simulink model "LHC_18kW_v0"  (R2015a)
settings: Solver=ode15s  StartTime=0.0  StopTime=10000  RelTol=1e-3
libraries: simCryogenics_lib x24, nesl_utility x16
settings Model: Creator=SK248285  LastModifiedBy=FB229602
settings SimscapeCC: SimscapeLogType=all  SimscapeLogLimitData=off

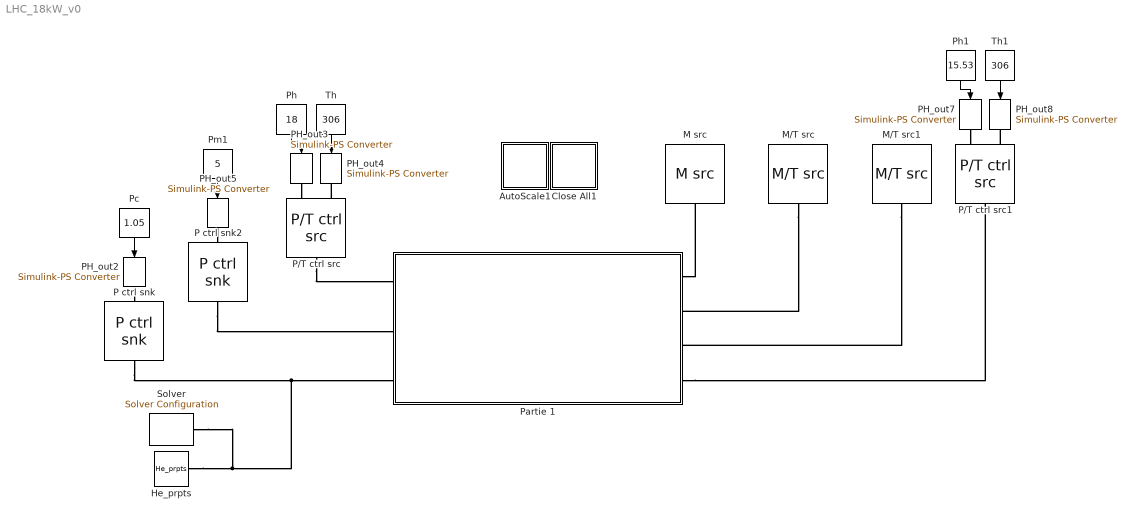
== system LHC_18kW_v0 ==
  AutoScale1 : Subsystem
      settings: OpenFcn=|
      | set(0, 'showhiddenhandles', 'on')
      | 
      | scope = findobj(0, 'Tag', 'SIMULINK_SIMSCOPE_FIGURE');
      | 
      | for i=1:length(scope)
      |   simscope('ScopeBar', 'ActionIcon', 'Find',     scope(i))
      | end
      | 
      | set(0, 'showhiddenhandles', 'off')
      mask Display: disp('Auto\nScale\nScope')
  Close All1 : Subsystem
      settings: OpenFcn=|
      | set(0, 'showhiddenhandles', 'on')
      | scope = findobj(0, 'Tag','SIMULINK_SIMSCOPE_FIGURE');
      | close(scope)
      | set(0, 'showhiddenhandles', 'off')
      mask Display: disp('Close\nAll\nScope')
  He_prpts : simCryogenics_lib/Utilities/He_prpts  P_min=0.1 bar  T_min=50 K  T_max=320 K  P_max=20 bar  Mol=4.0026 * 10 ^ (- 3) kg/mol
  M src : simCryogenics_lib/Sources_Sinks/M src  M=1 kg/s
  M/T src : simCryogenics_lib/Sources_Sinks/M//T src  M=0.350 kg/s  T=89 K
  M/T src1 : simCryogenics_lib/Sources_Sinks/M//T src  M=0.650 kg/s  T=89 K
  P ctrl snk : simCryogenics_lib/Sources_Sinks/P ctrl snk
  P ctrl snk2 : simCryogenics_lib/Sources_Sinks/P ctrl snk
  P/T ctrl src : simCryogenics_lib/Sources_Sinks/P//T ctrl src
  P/T ctrl src1 : simCryogenics_lib/Sources_Sinks/P//T ctrl src
  PH_out{2..3,5,7} (4 alike) : nesl_utility/Simulink-PS Converter  PhysicalDomain=network_engine_domain  SubClassName=ps_input  LeftPortType=input  RightPortType=output  PseudoPeriodic=off  Frequencies=[]  NoiseDistribution=none  NoiseParameters=[]  Unit=bar  AffineConversion=off  InputFiltering=off  SimscapeFilterOrder=1  InputFilterTimeConstant=0.001  UdotUserProvided=1
  PH_out4 : nesl_utility/Simulink-PS Converter  PhysicalDomain=network_engine_domain  SubClassName=ps_input  LeftPortType=input  RightPortType=output  PseudoPeriodic=off  Frequencies=[]  NoiseDistribution=none  NoiseParameters=[]  Unit=K  AffineConversion=off  InputFiltering=off  SimscapeFilterOrder=1  InputFilterTimeConstant=0.001  UdotUserProvided=1
  PH_out8 : nesl_utility/Simulink-PS Converter  PhysicalDomain=network_engine_domain  SubClassName=ps_input  LeftPortType=input  RightPortType=output  PseudoPeriodic=off  Frequencies=[]  NoiseDistribution=none  NoiseParameters=[]  Unit=K  AffineConversion=off  InputFiltering=off  SimscapeFilterOrder=1  InputFilterTimeConstant=0.001  UdotUserProvided=1
  Partie 1 : Subsystem
  Pc : Constant  Value=1.05
  Ph : Constant  Value=18
  Ph1 : Constant  Value=15.53
  Pm1 : Constant  Value=5
  Solver : nesl_utility/Solver Configuration  PhysicalDomain=network_engine_domain  SubClassName=solver  LeftPortType=input  RightPortType=generic  Accelerate=off  Tones=[]  Harmonics=[]  SimulateNoise=off  Profile=off  UseLocalSampling=off  EnableSwitchedLinearOptims=on  FrequencyDomain=off  UseCCode=off  RelTol=0.001  AbsTol=1e-06  MinStep=1e-09  ToWorkspace=off  RevertToSquareIcSolve=off  NumHomotopyIterations=100  DoDC=off  ResidualTolerance=1e-09  UseLocalSolver=off  LocalSolverChoice=NE_BACKWARD_EULER_ADVANCER  LocalSolverSampleTime=0.001  DoFixedCost=off  MaxNonlinIter=3  MaxModeIter=2  LinearAlgebra=Sparse  DelaysMemoryBudget=1024  AutomaticFiltering=on  FilteringTimeConstant=0.001
  Th : Constant  Value=306
  Th1 : Constant  Value=306
  wires:
  Th/1 -> PH_out4/1
  Ph/1 -> PH_out3/1
  Pc/1 -> PH_out2/1
  Pm1/1 -> PH_out5/1
  Th1/1 -> PH_out8/1
  Ph1/1 -> PH_out7/1
  connections:
  PH_out3/RConn1 -- P/T ctrl src/LConn1
  P/T ctrl src/LConn2 -- PH_out4/RConn1
  PH_out2/RConn1 -- P ctrl snk/LConn1
  P/T ctrl src/RConn1 -- Partie 1/LConn1
  PH_out5/RConn1 -- P ctrl snk2/LConn1
  P ctrl snk2/RConn1 -- Partie 1/LConn2
  He_prpts/RConn1 -- Solver/RConn1 -- P ctrl snk/RConn1 -- Partie 1/LConn3
  P/T ctrl src1/LConn2 -- PH_out8/RConn1
  PH_out7/RConn1 -- P/T ctrl src1/LConn1
  Partie 1/RConn4 -- P/T ctrl src1/RConn1
  M/T src1/RConn1 -- Partie 1/RConn3
  M/T src/RConn1 -- Partie 1/RConn2
  Partie 1/RConn1 -- M src/RConn1

== system LHC_18kW_v0/AutoScale1 ==

== system LHC_18kW_v0/Close All1 ==

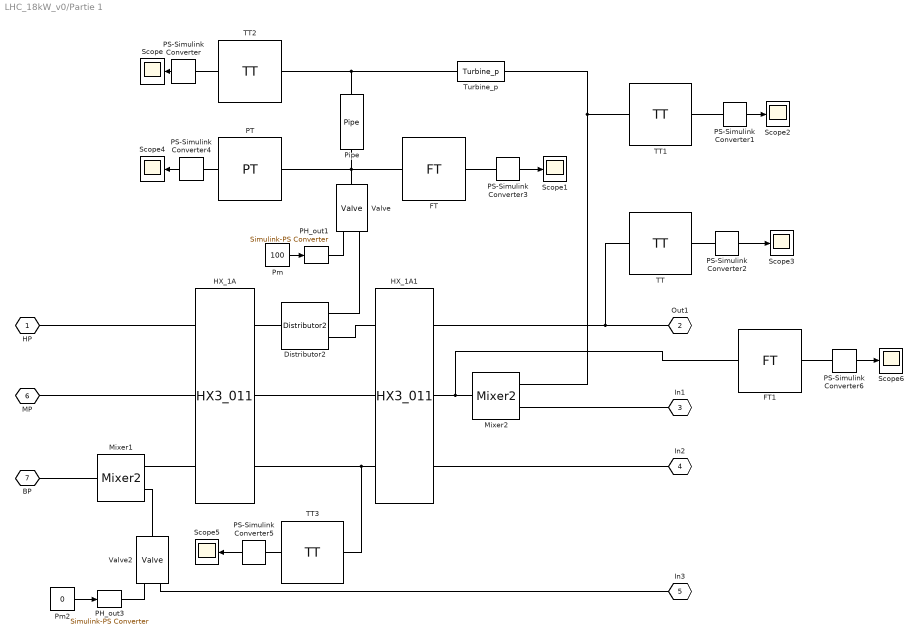
== system LHC_18kW_v0/Partie 1 ==
  Distributor2 : simCryogenics_lib/Elements/Distributor2
  FT : simCryogenics_lib/Sensors/FT
  FT1 : simCryogenics_lib/Sensors/FT
  HX_1A : simCryogenics_lib/Elements/HX3_011  N=10  Vh=1 m^3  Vm=1 m^3  Vc=1 m^3  M=1000 kg  Kh=0 s*bar/kg  Km=0 s*bar/kg  Kc=0 s*bar/kg  hh_m=5.0638e+04 J/s/K  hh_c=5.0638e+04 J/s/K  hm_c=1 J/s/K  Th0=306 K  Ph0=18 bar  Mh0=1 kg/s  Tm0=198 K  Pm0=5 bar  Mm0=0.5 kg/s  Tc0=198 K  Pc0=1.05 bar  Mc0=0.5 kg/s  sensh=0  sensm=1  sensc=1
  HX_1A1 : simCryogenics_lib/Elements/HX3_011  N=10  Vh=1 m^3  Vm=1 m^3  Vc=1 m^3  M=1000 kg  Kh=0 s*bar/kg  Km=0 s*bar/kg  Kc=0 s*bar/kg  hh_m=1e5 J/s/K  hh_c=1e5 J/s/K  hm_c=1 J/s/K  Th0=200 K  Ph0=18 bar  Mh0=1 kg/s  Tm0=89 K  Pm0=5 bar  Mm0=0.5 kg/s  Tc0=89 K  Pc0=1.05 bar  Mc0=0.5 kg/s  sensh=0  sensm=1  sensc=1
  Mixer1 : simCryogenics_lib/Elements/Mixer2
  Mixer2 : simCryogenics_lib/Elements/Mixer2
  PH_out1 : nesl_utility/Simulink-PS Converter  PhysicalDomain=network_engine_domain  SubClassName=ps_input  LeftPortType=input  RightPortType=output  PseudoPeriodic=off  Frequencies=[]  NoiseDistribution=none  NoiseParameters=[]  Unit=1  AffineConversion=off  InputFiltering=off  SimscapeFilterOrder=1  InputFilterTimeConstant=0.001  UdotUserProvided=1
  PH_out3 : nesl_utility/Simulink-PS Converter  PhysicalDomain=network_engine_domain  SubClassName=ps_input  LeftPortType=input  RightPortType=output  PseudoPeriodic=off  Frequencies=[]  NoiseDistribution=none  NoiseParameters=[]  Unit=1  AffineConversion=off  InputFiltering=off  SimscapeFilterOrder=1  InputFilterTimeConstant=0.001  UdotUserProvided=1
  PS-Simulink Converter{,1..6} (7 alike) : nesl_utility/PS-Simulink Converter  PhysicalDomain=network_engine_domain  SubClassName=ps_output  LeftPortType=input  RightPortType=output  PseudoPeriodic=off  Frequencies=[]  Unit=1  AffineConversion=off
  PT : simCryogenics_lib/Sensors/PT
  Pipe : simCryogenics_lib/Elements/Pipe  Vol=0.1 m^3  Ideal=0  P0=18 bar  T0=150 K
  Pm : Constant  Value=100
  Pm2 : Constant  Value=0
  Scope{,1..6} (7 alike) : Scope
      Scope1 settings: TimeRange=10000  YMin=0  YMax=0.4
      Scope2 settings: TimeRange=10000  YMin=60  YMax=160  SaveName=ScopeData2
      Scope3 settings: SaveName=ScopeData3
      Scope4 settings: TimeRange=10000  YMin=5.00151  YMax=5.00151  SaveName=ScopeData4
      Scope5 settings: TimeRange=10000  SaveName=ScopeData5
      Scope6 settings: TimeRange=10000  YMin=0  YMax=0.4  SaveName=ScopeData6
  TT{,1..3} (4 alike) : simCryogenics_lib/Sensors/TT
  Turbine_p : simCryogenics_lib/Elements/Turbine_p  A=1.2931e-04 m^2  D=0.05 m  Mass=0.02 kg  cst_eff=1  eta0=0.6  Tin0=150 K  Pin0=18 bar  Pout0=5 bar  N0=2500 1/s  Q0=0 W  v0=0  I=0 kg*m^2  gamma_specify=off  gamma_priority=High  gamma=0  C_specify=off  C_priority=High  C=0  Z_specify=off  Z_priority=High  Z=0  Cp_specify=off  Cp_priority=High  Cp=0 kJ/kg/K  Sin_specify=off  Sin_priority=High  Sin=0 kJ/kg  T_specify=off  T_priority=High  T=0 K  HoutIs_specify=off  HoutIs_priority=High  HoutIs=0 kJ/kg  u1_specify=off  u1_priority=High  u1=0 m/s  c1_specify=off  c1_priority=High  c1=0 m/s  v_specify=off  v_priority=High  v=0  eta_specify=off  eta_priority=High  eta=0  N_specify=off  N_priority=High  N=0 rad/s  Q_specify=off  Q_priority=High  Q=0 W
  Valve : simCryogenics_lib/Elements/Valve  CVmax=50  ControlInputMin=0  ControlInputMax=100  Xt=0.86  Rv=10  lin_v=0  lim_v=0  K=2.4e-5 m^1.50000*kg^0.50000/s/bar^0.50000  Cmd_specify=off  Cmd_priority=High  Cmd=0  gamma_specify=off  gamma_priority=High  gamma=0  rho_specify=off  rho_priority=High  rho=0 kg/m^3  Xc_specify=off  Xc_priority=High  Xc=0  X_specify=off  X_priority=High  X=0  Y_specify=off  Y_priority=High  Y=0  CV_specify=off  CV_priority=High  CV=0
  Valve2 : simCryogenics_lib/Elements/Valve  CVmax=3.2  ControlInputMin=0  ControlInputMax=100  Xt=0.86  Rv=10  lin_v=0  lim_v=0  K=2.4e-5 m^1.50000*kg^0.50000/s/bar^0.50000  Cmd_specify=off  Cmd_priority=High  Cmd=0  gamma_specify=off  gamma_priority=High  gamma=0  rho_specify=off  rho_priority=High  rho=0 kg/m^3  Xc_specify=off  Xc_priority=High  Xc=0  X_specify=off  X_priority=High  X=0  Y_specify=off  Y_priority=High  Y=0  CV_specify=off  CV_priority=High  CV=0
  HP : PMIOPort  Port=1  Side=Left
  Out1 : PMIOPort  Port=2  Side=Right
  In1 : PMIOPort  Port=3  Side=Right
  In2 : PMIOPort  Port=4  Side=Right
  In3 : PMIOPort  Port=5  Side=Right
  MP : PMIOPort  Port=6  Side=Left
  BP : PMIOPort  Port=7  Side=Left
  wires:
  Pm/1 -> PH_out1/1
  Pm2/1 -> PH_out3/1
  PS-Simulink Converter/1 -> Scope/1
  PS-Simulink Converter3/1 -> Scope1/1
  PS-Simulink Converter1/1 -> Scope2/1
  PS-Simulink Converter2/1 -> Scope3/1
  PS-Simulink Converter4/1 -> Scope4/1
  PS-Simulink Converter5/1 -> Scope5/1
  PS-Simulink Converter6/1 -> Scope6/1
  connections:
  Distributor2/RConn1 -- Valve/LConn2
  HX_1A1/LConn1 -- HX_1A/RConn1 -- TT3/LConn1
  Distributor2/LConn1 -- HX_1A/RConn3
  HX_1A1/LConn2 -- HX_1A/RConn2
  Distributor2/RConn2 -- HX_1A1/LConn3
  In2/RConn1 -- HX_1A1/RConn1
  Valve2/RConn1 -- Mixer1/LConn1
  Mixer2/LConn2 -- TT1/LConn1 -- Turbine_p/RConn1
  In1/RConn1 -- Mixer2/LConn1
  Mixer2/RConn1 -- FT1/LConn1 -- HX_1A1/RConn2
  HP/RConn1 -- HX_1A/LConn3
  BP/RConn1 -- Mixer1/RConn1
  MP/RConn1 -- HX_1A/LConn2
  Mixer1/LConn2 -- HX_1A/LConn1
  Turbine_p/LConn1 -- Pipe/RConn1 -- TT2/LConn1
  Pipe/LConn1 -- Valve/RConn1 -- PT/LConn1 -- FT/LConn1
  In3/RConn1 -- Valve2/LConn2
  PH_out3/RConn1 -- Valve2/LConn1
  Out1/RConn1 -- TT/LConn1 -- HX_1A1/RConn3
  PH_out1/RConn1 -- Valve/LConn1
  PS-Simulink Converter/LConn1 -- TT2/RConn1
  PS-Simulink Converter3/LConn1 -- FT/RConn1
  PS-Simulink Converter1/LConn1 -- TT1/RConn1
  PS-Simulink Converter2/LConn1 -- TT/RConn1
  PS-Simulink Converter4/LConn1 -- PT/RConn1
  PS-Simulink Converter5/LConn1 -- TT3/RConn1
  PS-Simulink Converter6/LConn1 -- FT1/RConn1
